simulink model "InnerOuter_Sim_newNav_flightgear_L2"  (Simulink 7.8)
settings: Solver=ode4  StartTime=0.0  StopTime=300  FixedStep=SampleT  RelTol=1e-3
InitFcn:
  | clc
  | innerOuterInit
  | launchFlightgear
values from neighbouring files (symbols this model uses):
  apSampleTime = 0.01    [innerOuterInit.m]
  FLIGHTGEAR_L2_RATE = 10    [launchFlightgear.m]
  SampleT = 0.005    [innerOuterInit.m]
  T = 0.01    [innerOuterInit.m]
undefined symbols (not defined in the file or in its folder): A1, Apolar, bankCommandLimit, baseHeight, BasePoint, baseTemp, CD0, chord, CL0, CLa, CLa_dot, Clb, ClDa, CLDe, CLDf, ClDr, clock, Clp, CLq, Clr, Cm0, Cma, CmDe, CmDf, Cmq, Cnb, CnDa, CnDr, Cnp, Cnr, compensatorOn, CYb, CYDr, da_failamp, da_failbias, da_failper, daL_fail, daR_fail, deg, DiscIntNeverNeededParam, dr_fail, dr_failamp, dr_failbias, dr_failper, Earth, elarm, Euler_0, F, gaind, getGSLocation, getWP, GS_location, Init_onlyOnce, Init_Reset, IPStar, ISA_g, Ixx, Iyy, Izz, L1OF ... (+38)
libraries: simulink x74, SLUGS_Library x41, aerolibconvert2 x24, dsPICdrivers x10, aerolibactuator x5, aerolibtransform2 x4, aerolibobsolete x3, dspmtrx3 x3, aerolibwind2 x2, aerolibfltsims x2, aerolibatmos2 x1, aerolibanimutils x1
(part 3 of 5)

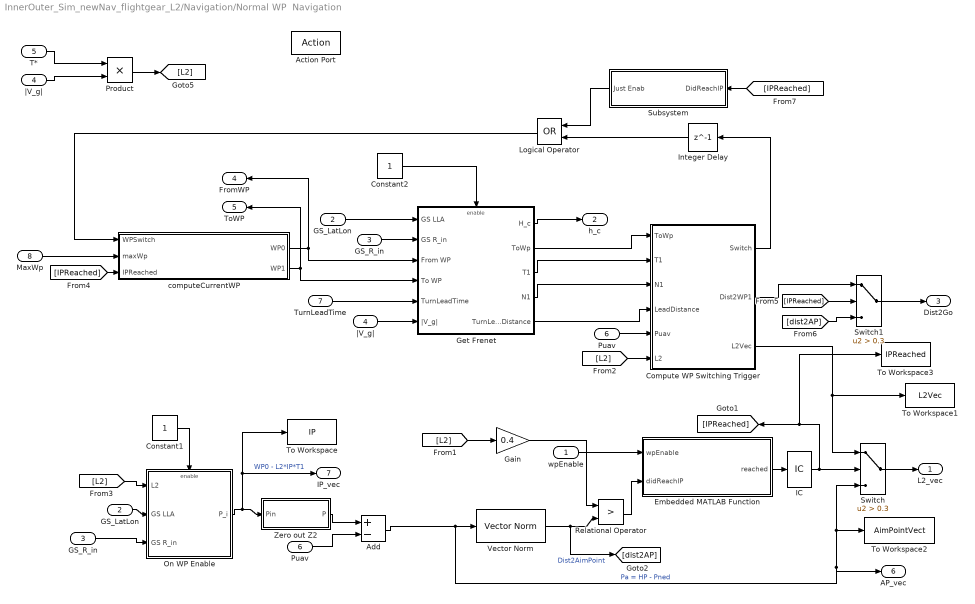
== system InnerOuter_Sim_newNav_flightgear_L2/Navigation/Normal WP  Navigation ==
  wpEnable : Inport
  GS_LatLon : Inport  Port=2
  GS_R_in : Inport  Port=3
  |V_g| : Inport  Port=4
  T* : Inport  Port=5
  Puav : Inport  Port=6
  TurnLeadTime : Inport  Port=7
  MaxWp : Inport  Port=8
  Action Port : ActionPort  ActionType=elseif
  Add : Sum  Inputs=+-
  Compute WP Switching Trigger : Subsystem
  Constant1 : Constant  OutDataTypeStr=boolean  SampleTime=0.01
  Constant2 : Constant  OutDataTypeStr=boolean  SampleTime=0.01
  Embedded MATLAB Function : MATLAB Function  TreatAsAtomicUnit=on
  "GS_LatLon " : InportShadow  Port=2
  "GS_R_in " : InportShadow  Port=3
  Gain : Gain  Gain=0.4
  Get Frenet : Subsystem
  IC : InitialCondition  Value=0
  Integer Delay : Delay  DelayLength=1  InitialCondition=1  InputProcessing=Inherited
  Logical Operator : Logic  Operator=OR  AllPortsSameDT=off  OutDataTypeStr=boolean
  On WP Enable : Subsystem  TreatAsAtomicUnit=on
  Product : Product  OutDataTypeStr=single  RndMeth=Zero
  "Puav " : InportShadow  Port=6
  Relational Operator : RelationalOperator  Operator=>  OutDataTypeStr=boolean
  Subsystem : Subsystem
  Switch : Switch  Criteria=u2 > Threshold  Threshold=0.3  ZeroCross=off
  Switch1 : Switch  Criteria=u2 > Threshold  Threshold=0.3  ZeroCross=off
  To Workspace : ToWorkspace  VariableName=IP  SampleTime=-1  SaveFormat=Array
  To Workspace1 : ToWorkspace  VariableName=L2Vec  SampleTime=-1  SaveFormat=Array
  To Workspace2 : ToWorkspace  VariableName=AimPointVect  SampleTime=-1  SaveFormat=Array
  To Workspace3 : ToWorkspace  VariableName=IPReached  SampleTime=-1  SaveFormat=Array
  Vector Norm : SLUGS_Library/Vector Norm
  Zero out Z2 : MATLAB Function  TreatAsAtomicUnit=on
  computeCurrentWP : MATLAB Function  TreatAsAtomicUnit=on
  "|V_g| " : InportShadow  Port=4
  L2_vec : Outport
  h_c : Outport  Port=2
  Dist2Go : Outport  Port=3
  FromWP : Outport  Port=4  InitialOutput=[1]
  ToWP : Outport  Port=5  InitialOutput=[2]
  AP_vec : Outport  Port=6
  IP_vec : Outport  Port=7
  wires:
  Get Frenet/1(H_c) -> h_c/1
  Constant2/1 -> Get Frenet/Enable
  Constant1/1 -> On WP Enable/Enable
  [IPReached] -> Subsystem/1(DidReachIP)
  Subsystem/1(Just Enab) -> Logical Operator/1
  Integer Delay/1 -> Logical Operator/2
  Logical Operator/1 -> computeCurrentWP/1(WPSwitch)
  [dist2AP] -> Switch1/3
  Switch1/1 -> Dist2Go/1
  Compute WP Switching Trigger/2(Dist2WP1) -> Switch1/1
  [IPReached] -> Switch1/2
  [IPReached] -> computeCurrentWP/3(IPReached)
  wpEnable/1 -> Embedded MATLAB Function/1(wpEnable)
  T*/1 -> Product/1
  |V_g|/1 -> Product/2
  Product/1 -> [L2]
  [L2] -> On WP Enable/1(L2)
  GS_LatLon/1 -> On WP Enable/2(GS LLA)
  GS_R_in/1 -> On WP Enable/3(GS R_in)
  On WP Enable/1(P_i) -> Zero out Z2/1(Pin), To Workspace/1, IP_vec/1  "WP0 - L2*IP*T1"
  Zero out Z2/1(P) -> Add/1
  Add/1 -> Vector Norm/1, Switch/3, To Workspace2/1, AP_vec/1  "Pa = HP - Pned"
  [L2] -> Gain/1
  Gain/1 -> Relational Operator/1
  Vector Norm/1 -> [dist2AP], Relational Operator/2  "Dist2AimPoint"
  Relational Operator/1 -> Embedded MATLAB Function/2(didReachIP)
  Switch/1 -> L2_vec/1
  Embedded MATLAB Function/1(reached) -> IC/1
  "GS_LatLon "/1 -> Get Frenet/1(GS LLA)
  "GS_R_in "/1 -> Get Frenet/2(GS R_in)
  Get Frenet/2(ToWp) -> Compute WP Switching Trigger/1(ToWp)
  Get Frenet/3(T1) -> Compute WP Switching Trigger/2(T1)
  Puav/1 -> Compute WP Switching Trigger/5(Puav)
  "Puav "/1 -> Add/2
  "|V_g| "/1 -> Get Frenet/6(|V_g|)
  TurnLeadTime/1 -> Get Frenet/5(TurnLeadTime)
  Get Frenet/5(TurnLeadDistance) -> Compute WP Switching Trigger/4(LeadDistance)
  Get Frenet/4(N1) -> Compute WP Switching Trigger/3(N1)
  Compute WP Switching Trigger/3(L2Vec) -> Switch/1, To Workspace1/1
  Compute WP Switching Trigger/1(Switch) -> Integer Delay/1
  computeCurrentWP/1(WP0) -> FromWP/1, Get Frenet/3(From WP)
  computeCurrentWP/2(WP1) -> ToWP/1, Get Frenet/4(To WP)
  MaxWp/1 -> computeCurrentWP/2(maxWp)
  [L2] -> Compute WP Switching Trigger/6(L2)
  IC/1 -> [IPReached], To Workspace3/1, Switch/2

== system InnerOuter_Sim_newNav_flightgear_L2/Navigation/RTB/Follow Mobile Navigation ==
  Mobile Location : Inport
  Follow Mobile? : Inport  Port=2
  MidLvl h_c : Inport  Port=3
  GS LatLon : Inport  Port=4
  GS R : Inport  Port=5
  Puav : Inport  Port=6
  Action Port : ActionPort  ActionType=then
  Compute Mobile Location : Subsystem  TreatAsAtomicUnit=on
  Constant : Constant  Value=[0 0 0]  OutDataTypeStr=single
  RTB : Constant  Value=0  OutDataTypeStr=uint8
  RTB1 : Constant  Value=0  OutDataTypeStr=uint8
  Simple Predictor : Subsystem
  Subtract : Sum  Inputs=+-
  Switch : Switch  Threshold=0.3
  To Workspace : ToWorkspace  VariableName=BP  SampleTime=-1  SaveFormat=Array
  Vector Norm : SLUGS_Library/Vector Norm
  Zero out Z1 : MATLAB Function  TreatAsAtomicUnit=on
  L2_vec : Outport
  h_c : Outport  Port=2
  Dist2Go : Outport  Port=3
  FromWP : Outport  Port=4  InitialOutput=[0]
  ToWP : Outport  Port=5  InitialOutput=[0]
  wires:
  RTB1/1 -> ToWP/1
  RTB/1 -> FromWP/1
  Vector Norm/1 -> Dist2Go/1
  Constant/1 -> Switch/3
  Compute Mobile Location/1(XYZ) -> Switch/1
  Follow Mobile?/1 -> Compute Mobile Location/Enable, Switch/2
  GS LatLon/1 -> Compute Mobile Location/2(GS LLA)
  GS R/1 -> Compute Mobile Location/3(GS R)
  Mobile Location/1 -> Compute Mobile Location/1("Lat, Lon")
  Simple Predictor/1(Predicted Bp) -> L2_vec/1
  Switch/1 -> Zero out Z1/1(Pin)
  Subtract/1 -> Vector Norm/1, Simple Predictor/1(Base Point), To Workspace/1
  Puav/1 -> Subtract/2
  Zero out Z1/1(P) -> Subtract/1
  MidLvl h_c/1 -> h_c/1

== system InnerOuter_Sim_newNav_flightgear_L2/Navigation/Recent Enable ==
  WP Fly : Inport
  Grab Upon Enable : Subsystem  TreatAsAtomicUnit=on
  IC1 : InitialCondition  Value=0
  IC2 : InitialCondition
  Subsystem : Subsystem
  WPEnable : Outport
  "GS, Lat Lon" : Outport  Port=2
  GS R_in : Outport  Port=3
  GS Alt (m) : Outport  Port=4
  wires:
  Grab Upon Enable/3(GS Altitude (m)) -> GS Alt (m)/1
  IC2/1 -> Grab Upon Enable/Enable
  IC1/1 -> Subsystem/1(WP Fly)
  Subsystem/1(Just Enab) -> IC2/1, WPEnable/1
  WP Fly/1 -> IC1/1
  Grab Upon Enable/1("GS, Lon, Lat") -> "GS, Lat Lon"/1
  Grab Upon Enable/2(GS R_in) -> GS R_in/1

== system InnerOuter_Sim_newNav_flightgear_L2/PT Unit (Vlad) /LPF the Euler and Construct Matrix ==
  Euler : Inport
  Euler Angles to  Direction Cosine Matrix : aerolibobsolete/Euler Angles to  Direction Cosine Matrix
  Terminator : Terminator
  "Tustin Lowpass, Auto Initial Condition1" : Subsystem  mask(Tustin1stOrderLowpassAutoInitialCondition){f=75, T=T}
      mask prompts: f "Lowpass Frequency"; T "Sample Time"
      mask help: Takes a 3db rolloff frequency (in Hz, NOT radians/s) and a sample time. Performs a symbolic Tustin conversion and implements in a discrete filter. The initial output of the filter is set by the first sample.
      mask Help: Enter the desired 3db rolloff frequency in Hz and the sample time. Initial conditions are sampled automatically.
      mask Display: fprintf('%.2f Hz lowpass',f)
  "Tustin Lowpass, Auto Initial Condition2" : Subsystem  mask(Tustin1stOrderLowpassAutoInitialCondition){f=75, T=T}
      mask prompts: f "Lowpass Frequency"; T "Sample Time"
      mask help: Takes a 3db rolloff frequency (in Hz, NOT radians/s) and a sample time. Performs a symbolic Tustin conversion and implements in a discrete filter. The initial output of the filter is set by the first sample.
      mask Help: Enter the desired 3db rolloff frequency in Hz and the sample time. Initial conditions are sampled automatically.
      mask Display: fprintf('%.2f Hz lowpass',f)
  "Tustin Lowpass, Auto Initial Condition3" : Subsystem  mask(Tustin1stOrderLowpassAutoInitialCondition){f=75, T=T}
      mask prompts: f "Lowpass Frequency"; T "Sample Time"
      mask help: Takes a 3db rolloff frequency (in Hz, NOT radians/s) and a sample time. Performs a symbolic Tustin conversion and implements in a discrete filter. The initial output of the filter is set by the first sample.
      mask Help: Enter the desired 3db rolloff frequency in Hz and the sample time. Initial conditions are sampled automatically.
      mask Display: fprintf('%.2f Hz lowpass',f)
  "[a b c]" : Demux  Outputs=3
  myMux Fun5 : MATLAB Function  TreatAsAtomicUnit=on
  Rfg2b : Outport
  wires:
  myMux Fun5/1(y) -> Terminator/1
  Euler/1 -> Euler Angles to  Direction Cosine Matrix/1, "[a b c]"/1
  "[a b c]"/3 -> "Tustin Lowpass, Auto Initial Condition3"/1(In1)
  "[a b c]"/2 -> "Tustin Lowpass, Auto Initial Condition1"/1(In1)
  "[a b c]"/1 -> "Tustin Lowpass, Auto Initial Condition2"/1(In1)
  "Tustin Lowpass, Auto Initial Condition3"/1(Out1) -> myMux Fun5/3(u3)
  "Tustin Lowpass, Auto Initial Condition1"/1(Out1) -> myMux Fun5/2(u2)
  "Tustin Lowpass, Auto Initial Condition2"/1(Out1) -> myMux Fun5/1(u1)
  Euler Angles to  Direction Cosine Matrix/1 -> Rfg2b/1

== system InnerOuter_Sim_newNav_flightgear_L2/Simple Car Model/Heading/Speed to Velocity ==
  Heading : Inport
  Speed : Inport  Port=2
  Add : Sum  Inputs=+-
  Angle Conversion : aerolibconvert2/Angle Conversion  IU=deg  OU=rad
  Divide : Product
  Divide1 : Product
  Low pass the  change of direction : Subsystem  mask(Tustin1stOrderLowpassAutoInitialCondition){f=0.05, T=apSampleTime}
      mask prompts: f "Lowpass Frequency"; T "Sample Time"
      mask help: Takes a 3db rolloff frequency (in Hz, NOT radians/s) and a sample time. Performs a symbolic Tustin conversion and implements in a discrete filter. The initial output of the filter is set by the first sample.
      mask Help: Enter the desired 3db rolloff frequency in Hz and the sample time. Initial conditions are sampled automatically.
      mask Display: fprintf('%.2f Hz lowpass',f)
  Mux : Mux  Inputs=3
  Rate Transition1 : RateTransition  OutPortSampleTime=apSampleTime
  Rate Transition2 : RateTransition  OutPortSampleTime=apSampleTime
  Speed1 : Constant  Value=0
  Speed2 : Constant  Value=450*pi/180  SampleTime=0.01
  Trigonometric Function : Trigonometry  Operator=cos
  Trigonometric Function1 : Trigonometry
  Velocity : Outport
  wires:
  Speed1/1 -> Mux/3
  Speed2/1 -> Add/1
  Add/1 -> Trigonometric Function/1, Trigonometric Function1/1  "alpha"
  Trigonometric Function/1 -> Divide/1
  Speed/1 -> Rate Transition2/1
  Divide/1 -> Mux/1
  Angle Conversion/1 -> Add/2
  Divide1/1 -> Mux/2
  Trigonometric Function1/1 -> Divide1/2
  Low pass the  change of direction/1(Out1) -> Angle Conversion/1
  Heading/1 -> Rate Transition1/1
  Mux/1 -> Velocity/1
  Rate Transition1/1 -> Low pass the  change of direction/1(In1)
  Rate Transition2/1 -> Divide1/1, Divide/2

== system InnerOuter_Sim_newNav_flightgear_L2/Simple Car Model/Simple Car Model ==
  Velocity : Inport
  Constant13 : Constant  Value=BasePoint  OutDataTypeStr=single
  Data Type Conversion : DataTypeConversion  OutDataTypeStr=single
  Data Type Conversion1 : DataTypeConversion  OutDataTypeStr=single
  Discrete-Time Integrator : DiscreteIntegrator  InitialConditionSource=external  SampleTime=0.01  ICPrevOutput=DiscIntNeverNeededParam  ICPrevScaledInput=DiscIntNeverNeededParam
  p_cg : Outport
  wires:
  Velocity/1 -> Data Type Conversion1/1
  Constant13/1 -> Discrete-Time Integrator/2
  Discrete-Time Integrator/1 -> Data Type Conversion/1
  Data Type Conversion/1 -> p_cg/1
  Data Type Conversion1/1 -> Discrete-Time Integrator/1

== system InnerOuter_Sim_newNav_flightgear_L2/6DOF Model/Plant/6-DOF EOM ==
  "[F,M]" : Inport
  Vb Corr : Inport  Port=2
  Angular Rates : Integrator  InitialCondition=PQR_0'
  Demux1 : Demux  Outputs=2
  Euler Angles : Integrator  InitialCondition=Euler_0
  Get Euler Dot : Subsystem
      mask Display:
      | port_label('input', 1, 'p, q, r')
      | port_label('input', 2, 'Euler')
      | port_label('output', 1, 'Euler_dot')
  Mux : Mux  Inputs=[3;3]
  NED2NEU : Gain  Gain=[1 0 0;0 1 0;0 0 -1]  Multiplication=Matrix(K*u)  SaturateOnIntegerOverflow=on  OutDataTypeStr=Inherit: Same as input  ParamDataTypeStr=Inherit: Same as input
  Position : Integrator  InitialCondition=Pos_0'
  RB2L * Vb : Product  Multiplication=Matrix(*)  SaturateOnIntegerOverflow=on  InputSameDT=on  OutDataTypeStr=Inherit: Same as first input
  RB2LTP : Subsystem
  Velocities Body : Integrator  InitialCondition=Vb_0'
  "[V1,2,3,W1,2,3]" : Subsystem
  X,Y,Z (LTP) : Outport
  "Vx, Vy, Vz" : Outport  Port=2
  Euler : Outport  Port=3
  "p, q, r" : Outport  Port=4
  Vb : Outport  Port=5
  Ab meas : Outport  Port=6
  Euler_dot : Outport  Port=7
  wires:
  "[V1,2,3,W1,2,3]"/1("Acc_meas ") -> Ab meas/1
  Euler Angles/1 -> "[V1,2,3,W1,2,3]"/2(Euler), Get Euler Dot/2(Euler), Euler/1, RB2LTP/1(Euler)
  Demux1/1 -> Velocities Body/1
  "[V1,2,3,W1,2,3]"/2(V*dot) -> Demux1/1
  Demux1/2 -> Angular Rates/1
  "[F,M]"/1 -> "[V1,2,3,W1,2,3]"/1("[F ; M]")
  RB2LTP/1(Rot) -> RB2L * Vb/1
  Velocities Body/1 -> Vb/1, RB2L * Vb/2
  Mux/1 -> "[V1,2,3,W1,2,3]"/3(V*)
  Position/1 -> X,Y,Z (LTP)/1
  Angular Rates/1 -> Get Euler Dot/1(p,q,r), Mux/2, "p, q, r"/1
  RB2L * Vb/1 -> NED2NEU/1, "Vx, Vy, Vz"/1  "NED"
  NED2NEU/1 -> Position/1
  Get Euler Dot/1(Euler_dot) -> Euler Angles/1, Euler_dot/1
  Vb Corr/1 -> Mux/1

== system InnerOuter_Sim_newNav_flightgear_L2/6DOF Model/Plant/Engine Model ==
  dt : Inport
  Vmag : Inport  Port=2
  Constant4 : Constant  Value=0
  Get To1 : Subsystem
  Mux : Mux  Inputs=2
  Mux1 : Mux  Inputs=3
  Thrust Available (lbs) : Fcn  Expr=u(1) - 0.047*sqrt(u(1))*u(2)
  kg2N : Gain  Gain=ISA_g  SaturateOnIntegerOverflow=on  OutDataTypeStr=Inherit: Same as input  ParamDataTypeStr=Inherit: Same as input
  lbs2kg : Gain  Gain=0.45359237  SaturateOnIntegerOverflow=on  OutDataTypeStr=Inherit: Same as input  ParamDataTypeStr=Inherit: Same as input
  Thrust : Outport
  wires:
  dt/1 -> Get To1/1(dt)
  Get To1/1(To) -> Mux/1
  Mux/1 -> Thrust Available (lbs)/1
  Thrust Available (lbs)/1 -> lbs2kg/1
  Vmag/1 -> Mux/2
  Mux1/1 -> Thrust/1
  lbs2kg/1 -> kg2N/1
  Constant4/1 -> Mux1/2, Mux1/3
  kg2N/1 -> Mux1/1

== system InnerOuter_Sim_newNav_flightgear_L2/6DOF Model/Plant/Forces and Moments ==
  "Wind {E}" : Inport
  Rho : Inport  Port=2
  "de, deg" : Inport  Port=3
  daL,deg : Inport  Port=4
  daR,deg : Inport  Port=5
  "dr, deg" : Inport  Port=6
  "df, deg" : Inport  Port=7
  "Vx, Vy, Vz " : Inport  Port=8
  Euler : Inport  Port=9  PortDimensions=3
  p,q,r : Inport  Port=10
  Alpha/Beta : Subsystem
  Body Frame F & M : Subsystem
  Get Grav Force in Body : Subsystem
  Gravitational Force : Constant  Value=[0 0 mass*ISA_g]  VectorParams1D=off
  NED(u)2b : Subsystem
  Sum : Sum  Inputs=|++  SaturateOnIntegerOverflow=on
  Vair : Sum  Inputs=+-  SaturateOnIntegerOverflow=on  InputSameDT=on  OutDataTypeStr=Inherit: Same as first input
  Airspeed : Outport
  Forces : Outport  Port=2
  Moments : Outport  Port=3
  Vb Corr : Outport  Port=4
  q : Outport  Port=5
  wires:
  Get Grav Force in Body/1(Grav Force (Body)) -> Sum/2
  Alpha/Beta/5(q) -> q/1
  "Vx, Vy, Vz "/1 -> Vair/1
  Vair/1 -> NED(u)2b/1(V w)
  Euler/1 -> NED(u)2b/2(Euler), Get Grav Force in Body/1(Euler)
  Rho/1 -> Alpha/Beta/2(Rho)
  NED(u)2b/1(Vb Corr) -> Alpha/Beta/1("Vx, Vy, Vz (Body)"), Vb Corr/1
  Body Frame F & M/2(M_b) -> Moments/1
  Gravitational Force/1 -> Get Grav Force in Body/2(Grav Force)
  Body Frame F & M/1(F_b) -> Sum/1
  Sum/1 -> Forces/1
  Alpha/Beta/3(qS) -> Body Frame F & M/3(qs)
  Alpha/Beta/4(Speed) -> Body Frame F & M/4(Airspeed), Airspeed/1
  "df, deg"/1 -> Body Frame F & M/9("df, deg")
  p,q,r/1 -> Body Frame F & M/10(p,q,r)
  Alpha/Beta/2("beta, deg") -> Body Frame F & M/2("Beta, deg")
  "dr, deg"/1 -> Body Frame F & M/8("dr, deg")
  daL,deg/1 -> Body Frame F & M/6("daL, deg")
  Alpha/Beta/1("alpha, deg") -> Body Frame F & M/1("Alpha, deg")
  "de, deg"/1 -> Body Frame F & M/5("de, deg")
  "Wind {E}"/1 -> Vair/2
  daR,deg/1 -> Body Frame F & M/7("daR, deg")

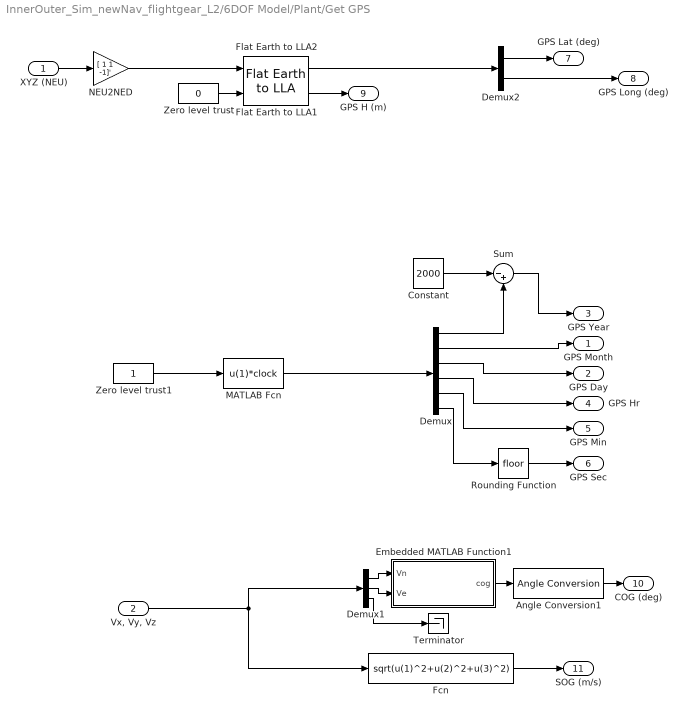
== system InnerOuter_Sim_newNav_flightgear_L2/6DOF Model/Plant/Get GPS ==
  XYZ (NEU) : Inport
  "Vx, Vy, Vz" : Inport  Port=2
  Angle Conversion1 : aerolibconvert2/Angle Conversion  IU=rad  OU=deg
  Constant : Constant  Value=2000
  Demux : Demux  Outputs=6
  Demux1 : Demux  Outputs=3
  Demux2 : Demux  Outputs=2
  Embedded MATLAB Function1 : MATLAB Function  TreatAsAtomicUnit=on
  Fcn : Fcn  Expr=sqrt(u(1)^2+u(2)^2+u(3)^2)
  Flat Earth to LLA1 : aerolibtransform2/Flat Earth to LLA  units=Metric (MKS)  ptype=Earth (WGS84)  F=1/298.257223563  R=6378137  LL0=GS_location(2:3)  psi=0
  Flat Earth to LLA2 : aerolibtransform2/Flat Earth to LLA  units=Metric (MKS)  ptype=Earth (WGS84)  F=1/298.257223563  R=6378137  LL0=GS_location(2:3)  psi=0
  MATLAB Fcn : MATLABFcn  MATLABFcn=u(1)*clock  OutputSignalType=real  SampleTime=SampleT
  NEU2NED : Gain  Gain=[ 1 1 -1]'  SaturateOnIntegerOverflow=on  OutDataTypeStr=Inherit: Same as input  ParamDataTypeStr=Inherit: Same as input
  Rounding Function : Rounding
  Sum : Sum  Inputs=|-+
  Terminator : Terminator
  Zero level trust : Constant  Value=0  SampleTime=SampleT
  Zero level trust1 : Constant  SampleTime=SampleT
  GPS Month : Outport
  GPS Day : Outport  Port=2
  GPS Year : Outport  Port=3
  GPS Hr : Outport  Port=4
  GPS Min : Outport  Port=5
  GPS Sec : Outport  Port=6
  GPS Lat (deg) : Outport  Port=7
  GPS Long (deg) : Outport  Port=8
  GPS H (m) : Outport  Port=9
  COG (deg) : Outport  Port=10
  SOG (m/s) : Outport  Port=11
  wires:
  NEU2NED/1 -> Flat Earth to LLA2/1
  Zero level trust/1 -> Flat Earth to LLA2/2
  XYZ (NEU)/1 -> NEU2NED/1
  Flat Earth to LLA2/1 -> Demux2/1
  Flat Earth to LLA2/2 -> GPS H (m)/1
  Zero level trust1/1 -> MATLAB Fcn/1
  MATLAB Fcn/1 -> Demux/1
  Demux/2 -> GPS Month/1
  Demux/3 -> GPS Day/1
  Demux/4 -> GPS Hr/1
  Demux/5 -> GPS Min/1
  Demux/6 -> Rounding Function/1
  Rounding Function/1 -> GPS Sec/1
  Demux2/1 -> GPS Lat (deg)/1
  Demux2/2 -> GPS Long (deg)/1
  Fcn/1 -> SOG (m/s)/1
  Demux1/1 -> Embedded MATLAB Function1/1(Vn)
  Demux1/2 -> Embedded MATLAB Function1/2(Ve)
  "Vx, Vy, Vz"/1 -> Demux1/1, Fcn/1
  Embedded MATLAB Function1/1(cog) -> Angle Conversion1/1
  Angle Conversion1/1 -> COG (deg)/1
  Demux/1 -> Sum/2
  Constant/1 -> Sum/1
  Sum/1 -> GPS Year/1
  Demux1/3 -> Terminator/1

== system InnerOuter_Sim_newNav_flightgear_L2/6DOF Model/Plant/ISA Atmosphere & Winds ==
  "X, Y, Z" : Inport
  Euler : Inport  Port=2
  Wind On : Inport  Port=3
  Airspeed : Inport  Port=4
  Add : Sum  Inputs=2
  Constant : Constant  Value=[ 0 0 0]
  Dryden Wind Turbulence Model  (Discrete (+q -r)) : aerolibwind2/Dryden Wind Turbulence Model  (Continuous (+q -r))  units=Metric (MKS)  spec=MIL-F-8785C  model=Discrete Dryden (+q -r)  W20=windBase*0.3  Wdeg=windDirTurb  TurbProb=10^-2 - Light  L_high=533.4  Wingspan=span  ts=0.005  Seed=[23341 23342 23343 23344]  T_on=on
  Euler Angles to  Direction Cosine Matrix1 : aerolibobsolete/Euler Angles to  Direction Cosine Matrix
  Get Z : Selector  InputPortWidth=3  IndexOptions=Index vector (dialog)  Indices=[3]  OutputSizes=[(-2)]
  Horizontal Wind Model : aerolibwind2/Horizontal Wind Model  units=Metric (MKS)  Vw_source=Internal  Vwind=windBase  W_source=Internal  Wdeg=windDirHor
  ISA Atmosphere Model1 : aerolibatmos2/ISA Atmosphere Model  custom=off  g=9.80665  gamma=1.4  R=287.0531  L=0.0065  h_trop=11000  h_strat=20000  rho0=1.225  P0=101325  T0=288.15
  Reduce Z Wind : Gain  Gain=[1 1 0.1]
  Rotate to E Frame : Product  Multiplication=Matrix(*)
  Scope : Scope
      settings: YMin=-1  YMax=13  SaveName=windData  DataFormat=Array
  Switch : Switch  Criteria=u2 > Threshold  Threshold=0.3
  Terminator1 : Terminator
  Transpose : dspmtrx3/Transpose  Hermitian=off  overflowFlag=off
  Unit Delay : UnitDelay  SampleTime=-1
  Rho : Outport
  "Wind, {E}" : Outport  Port=2
  AirPressure (Pa) : Outport  Port=3
  OAT (K) : Outport  Port=4
  wires:
  "X, Y, Z"/1 -> Get Z/1
  Get Z/1 -> ISA Atmosphere Model1/1, Dryden Wind Turbulence Model  (Discrete (+q -r))/1
  ISA Atmosphere Model1/4 -> Rho/1
  ISA Atmosphere Model1/1 -> OAT (K)/1
  ISA Atmosphere Model1/2 -> Terminator1/1
  ISA Atmosphere Model1/3 -> AirPressure (Pa)/1
  Euler/1 -> Euler Angles to  Direction Cosine Matrix1/1
  Euler Angles to  Direction Cosine Matrix1/1 -> Dryden Wind Turbulence Model  (Discrete (+q -r))/3, Horizontal Wind Model/1, Transpose/1  "RECEF2B"
  Airspeed/1 -> Unit Delay/1
  Add/1 -> Switch/1
  Unit Delay/1 -> Dryden Wind Turbulence Model  (Discrete (+q -r))/2
  Horizontal Wind Model/1 -> Add/2
  Switch/1 -> Rotate to E Frame/2
  Wind On/1 -> Switch/2
  Constant/1 -> Switch/3
  Transpose/1 -> Rotate to E Frame/1
  Rotate to E Frame/1 -> "Wind, {E}"/1, Scope/1
  Dryden Wind Turbulence Model  (Discrete (+q -r))/1 -> Reduce Z Wind/1
  Reduce Z Wind/1 -> Add/1

== system InnerOuter_Sim_newNav_flightgear_L2/6DOF Model/Plant/Magnetometer ==
  Euler : Inport
  LTP2B : dspmtrx3/Transpose  Hermitian=off  overflowFlag=off
  Mag Field in nT source:  http://www.ngdc.noaa.gov/geomagmodels/struts/calcIGRFWMM : Constant  Value=magField
  Product : Product  Multiplication=Matrix(*)  RndMeth=Zero
  RB2LTP : Subsystem
  "Mag, nT" : Outport
  wires:
  RB2LTP/1(Rot) -> LTP2B/1
  LTP2B/1 -> Product/1
  Mag Field in nT source:  http://www.ngdc.noaa.gov/geomagmodels/struts/calcIGRFWMM/1 -> Product/2
  Euler/1 -> RB2LTP/1(Euler)
  Product/1 -> "Mag, nT"/1

== system InnerOuter_Sim_newNav_flightgear_L2/6DOF Model/Plant/[0, pi] Wrap Around ==
  Euler : Inport
  Compare To Zero : simulink/Logic and Bit Operations/Compare To Zero  relop=>=  OutDataTypeStr=uint8  ZeroCross=off
  Logical Operator : Logic  Operator=NOT  AllPortsSameDT=off  OutDataTypeStr=boolean
  Merge : Merge
  Mux2 : Mux  Inputs=2
  Negative Yaw : Subsystem
  Positive Yaw : Subsystem
  Selector1 : Selector  InputPortWidth=3  IndexOptions=Index vector (dialog)  Indices=[1 2]  OutputSizes=1
  Selector2 : Selector  InputPortWidth=3  IndexOptions=Index vector (dialog)  Indices=[3]  OutputSizes=1
  Euler-Wrapped : Outport
  wires:
  Euler/1 -> Selector2/1, Selector1/1
  Selector1/1 -> Mux2/1
  Mux2/1 -> Euler-Wrapped/1
  Selector2/1 -> Compare To Zero/1, Positive Yaw/1(yaw), Negative Yaw/1(yaw)
  Compare To Zero/1 -> Positive Yaw/Enable, Logical Operator/1
  Logical Operator/1 -> Negative Yaw/Enable
  Merge/1 -> Mux2/2
  Positive Yaw/1(yaw_wr) -> Merge/1
  Negative Yaw/1(yaw_wr) -> Merge/2

== system InnerOuter_Sim_newNav_flightgear_L2/6DOF Model/Split Ailerons And Introduce Failures/Aileron Flaping Failure ==
  Pulse Generator1 : DiscretePulseGenerator  PulseType=Time based  Amplitude=da_failamp  Period=da_failper  PulseWidth=50
  Vair2 : Sum  Inputs=+++  SaturateOnIntegerOverflow=on  InputSameDT=on  OutDataTypeStr=Inherit: Same as first input
  da_failbias : Constant  Value=da_failbias
  da_failbias1 : Constant  Value=0
  "da, Fail, deg" : Outport
  wires:
  Pulse Generator1/1 -> Vair2/1
  da_failbias/1 -> Vair2/2
  da_failbias1/1 -> Vair2/3
  Vair2/1 -> "da, Fail, deg"/1

== system InnerOuter_Sim_newNav_flightgear_L2/6DOF Model/Split Ailerons And Introduce Failures/Rudder Failure ==
  Pulse Generator1 : DiscretePulseGenerator  PulseType=Time based  Amplitude=dr_failamp  Period=dr_failper  PulseWidth=50
  Vair2 : Sum  Inputs=+++  SaturateOnIntegerOverflow=on  InputSameDT=on  OutDataTypeStr=Inherit: Same as first input
  da_failbias : Constant  Value=dr_failbias
  da_failbias1 : Constant  Value=0
  "da, Fail, deg" : Outport
  wires:
  Vair2/1 -> "da, Fail, deg"/1
  da_failbias1/1 -> Vair2/3
  da_failbias/1 -> Vair2/2
  Pulse Generator1/1 -> Vair2/1

== system InnerOuter_Sim_newNav_flightgear_L2/BaroTest/Initial Baro Bias/Low Pass8 ==
  In1 : Inport
  Discrete Zero-Pole : DiscreteZeroPole  Zeros=zerosd  Poles=polesd  Gain=gaind  SampleTime=SampleTime
  Out1 : Outport
  wires:
  In1/1 -> Discrete Zero-Pole/1
  Discrete Zero-Pole/1 -> Out1/1

== system InnerOuter_Sim_newNav_flightgear_L2/L1 Output Feedback Controller With  Projection Operator/Control  Law/Compute Coef ==
  a : Inport
  Enable : EnablePort
  -T : Gain  Gain=-apSampleTime  SampleTime=apSampleTime
  1-c : Sum  Inputs=-+  OutDataTypeStr=single  SampleTime=apSampleTime
  Constant : Constant
  Subsystem11 : Subsystem  AncestorBlock=SLUGS_Library/Subsystem11
  b : Outport
  c : Outport  Port=2
  wires:
  a/1 -> -T/1
  1-c/1 -> b/1
  Constant/1 -> 1-c/2
  Subsystem11/1(exp(u)) -> c/1, 1-c/1  "c"
  -T/1 -> Subsystem11/1(u)

== system InnerOuter_Sim_newNav_flightgear_L2/L1 Output Feedback Controller With  Projection Operator/Control  Law/Detect Change ==
  Data : Inport
  Abs1 : Abs  SampleTime=apSampleTime
  Difference1 : simulink/Discrete/Difference  ICPrevInput=0.0  InputProcessing=Inherited  OutMin=[]  OutMax=[]  OutDataType=sfix(16)  OutScaling=2^-10  DoSatur=off
  Saturation1 : Saturate  UpperLimit=1  LowerLimit=0  SampleTime=apSampleTime
  change? : Outport
  wires:
  Saturation1/1 -> change?/1
  Data/1 -> Difference1/1
  Abs1/1 -> Saturation1/1
  Difference1/1 -> Abs1/1

== system InnerOuter_Sim_newNav_flightgear_L2/L1 Output Feedback Controller With  Projection Operator/Projection Operator/Enabled Subsystem ==
  In1 : Inport
  Enable : EnablePort
  Out1 : Outport
  wires:
  In1/1 -> Out1/1

== system InnerOuter_Sim_newNav_flightgear_L2/L1 Output Feedback Controller With  Projection Operator/Projection Operator/Enabled Subsystem1 ==
  y : Inport
  f_the : Inport  Port=2
  grad : Inport  Port=3
  Enable : EnablePort
  Constant : Constant  OutDataTypeStr=single
  Divide1 : Product  OutDataTypeStr=single
  Divide2 : Product  OutDataTypeStr=single
  Sign : Signum
  Subtract : Sum  Inputs=+-  OutDataTypeStr=single
  Out1 : Outport
  wires:
  Divide2/1 -> Out1/1
  y/1 -> Divide2/1
  Subtract/1 -> Divide2/2
  f_the/1 -> Divide1/1
  Constant/1 -> Subtract/1
  Sign/1 -> Divide1/2
  grad/1 -> Sign/1
  Divide1/1 -> Subtract/2

== system InnerOuter_Sim_newNav_flightgear_L2/L1 Output Feedback Controller With  Projection Operator/Projection Operator/Enabled Subsystem2 ==
  y : Inport
  f_the : Inport  Port=2
  grad : Inport  Port=3
  Enable : EnablePort
  Constant : Constant  OutDataTypeStr=single
  Divide1 : Product  OutDataTypeStr=single
  Divide2 : Product  OutDataTypeStr=single
  Sign : Signum
  Subtract : Sum  Inputs=+-  OutDataTypeStr=single
  Out1 : Outport
  wires:
  Divide1/1 -> Subtract/2
  grad/1 -> Sign/1
  Sign/1 -> Divide1/2
  Constant/1 -> Subtract/1
  f_the/1 -> Divide1/1
  Subtract/1 -> Divide2/2
  y/1 -> Divide2/1
  Divide2/1 -> Out1/1

== system InnerOuter_Sim_newNav_flightgear_L2/L1 Output Feedback Controller With  Projection Operator/Projection Operator/F(theta) ==
  Theta Max : Inport
  Eps 0 : Inport  Port=2
  Theta : Inport  Port=3
  Constant : Constant  Value=2  OutDataTypeStr=single
  Divide : Product  OutDataTypeStr=single
  Divide1 : Product  OutDataTypeStr=single
  Divide2 : Product  OutDataTypeStr=single
  Divide3 : Product  Inputs=*/  OutDataTypeStr=single
  Divide4 : Product  Inputs=/**  OutDataTypeStr=single
  Subtract : Sum  Inputs=+-  OutDataTypeStr=single
  "Theta " : InportShadow  Port=3
  f_theta : Outport
  dif_f_theta : Outport  Port=2
  wires:
  Divide4/1 -> dif_f_theta/1
  "Theta "/1 -> Divide4/2
  Constant/1 -> Divide4/3
  Divide3/1 -> f_theta/1
  Divide2/1 -> Divide4/1, Divide3/2
  Subtract/1 -> Divide3/1
  Eps 0/1 -> Divide2/2
  Divide1/1 -> Divide2/1, Subtract/2
  Divide/1 -> Subtract/1
  Theta Max/1 -> Divide1/1, Divide1/2
  Theta/1 -> Divide/2, Divide/1

== system InnerOuter_Sim_newNav_flightgear_L2/L1 Output Feedback Controller With  Projection Operator/State Predictor/Compute Coef ==
  a : Inport
  Enable : EnablePort
  -T : Gain  Gain=-apSampleTime  SampleTime=apSampleTime
  1-c : Sum  Inputs=-+  OutDataTypeStr=single
  Constant : Constant
  Subsystem11 : Subsystem  AncestorBlock=SLUGS_Library/Subsystem11
  b : Outport
  c : Outport  Port=2
  wires:
  -T/1 -> Subsystem11/1(u)
  Subsystem11/1(exp(u)) -> 1-c/1, c/1  "c"
  Constant/1 -> 1-c/2
  1-c/1 -> b/1
  a/1 -> -T/1

== system InnerOuter_Sim_newNav_flightgear_L2/L1 Output Feedback Controller With  Projection Operator/State Predictor/Detect Change ==
  Data : Inport
  Abs1 : Abs  SampleTime=apSampleTime
  Difference1 : simulink/Discrete/Difference  ICPrevInput=0.0  InputProcessing=Inherited  OutMin=[]  OutMax=[]  OutDataType=sfix(16)  OutScaling=2^-10  DoSatur=off
  Saturation1 : Saturate  UpperLimit=1  LowerLimit=0  SampleTime=apSampleTime
  change? : Outport
  wires:
  Difference1/1 -> Abs1/1
  Abs1/1 -> Saturation1/1
  Data/1 -> Difference1/1
  Saturation1/1 -> change?/1

== system InnerOuter_Sim_newNav_flightgear_L2/L1 Output Feedback Controller With  Projection Operator/Trapezoidal Integrator/Protect NaNs ==
  In1 : Inport
  Integer Delay3 : Delay  DelayLength=1  InputProcessing=Inherited  SampleTime=T
  Relational Operator2 : RelationalOperator  Operator===  OutDataTypeStr=uint(8)
  Switch3 : Switch  Criteria=u2 > Threshold  Threshold=0.3  SampleTime=.01
  Out1 : Outport
  wires:
  Integer Delay3/1 -> Switch3/3
  Switch3/1 -> Out1/1, Integer Delay3/1
  In1/1 -> Relational Operator2/2, Relational Operator2/1, Switch3/1
  Relational Operator2/1 -> Switch3/2

== system InnerOuter_Sim_newNav_flightgear_L2/L1 Output Feedback Controller With  Projection Operator/Trapezoidal Integrator/Protect NaNs1 ==
  In1 : Inport
  Integer Delay3 : Delay  DelayLength=1  InputProcessing=Inherited  SampleTime=T
  Relational Operator2 : RelationalOperator  Operator===  OutDataTypeStr=uint(8)
  Switch3 : Switch  Criteria=u2 > Threshold  Threshold=0.3  SampleTime=.01
  Out1 : Outport
  wires:
  Relational Operator2/1 -> Switch3/2
  In1/1 -> Switch3/1, Relational Operator2/1, Relational Operator2/2
  Switch3/1 -> Integer Delay3/1, Out1/1
  Integer Delay3/1 -> Switch3/3

== system InnerOuter_Sim_newNav_flightgear_L2/Navigation/Circle Navigation/Get SP Location ==
  GS LLA : Inport
  GS R_in : Inport  Port=2
  ISR Location : Inport  Port=3
  Demux : Demux  Outputs=3
  Geod2LTP : SLUGS_Library/Navigation/Geod2LTP
  Integer Delay1 : Delay  DelayLength=1  InputProcessing=Inherited
  Selector : Selector  InputPortWidth=3  IndexOptions=Index vector (dialog)  Indices=[3]  OutputSizes=1
  Zero out Z2 : MATLAB Function  TreatAsAtomicUnit=on
  Hc : Outport
  SP : Outport  Port=2
  wires:
  Integer Delay1/1 -> Hc/1
  Selector/1 -> Integer Delay1/1
  Zero out Z2/1(P) -> SP/1
  Geod2LTP/1 -> Selector/1, Zero out Z2/1(Pin)
  GS LLA/1 -> Geod2LTP/1
  Demux/3 -> Geod2LTP/5
  Demux/2 -> Geod2LTP/4
  Demux/1 -> Geod2LTP/3
  GS R_in/1 -> Geod2LTP/2
  ISR Location/1 -> Demux/1

== system InnerOuter_Sim_newNav_flightgear_L2/Navigation/Circle Navigation/Inside the Circle,  Keep Straight until  intersection ==
  ISR Loc : Inport
  R : Inport  Port=2
  Puav : Inport  Port=3
  Action Port : ActionPort  ActionType=elseif
  Compute Head of Circle : MATLAB Function  TreatAsAtomicUnit=on
  RTB1 : Constant  OutDataTypeStr=uint8
  Subtract : Sum  Inputs=+-  OutDataTypeStr=single
  L2 Vec : Outport
  Mode : Outport  Port=2
  wires:
  RTB1/1 -> Mode/1
  R/1 -> Compute Head of Circle/1(R)
  ISR Loc/1 -> Compute Head of Circle/2(ISR)
  Compute Head of Circle/1(topCoord) -> Subtract/1
  Puav/1 -> Subtract/2
  Subtract/1 -> L2 Vec/1

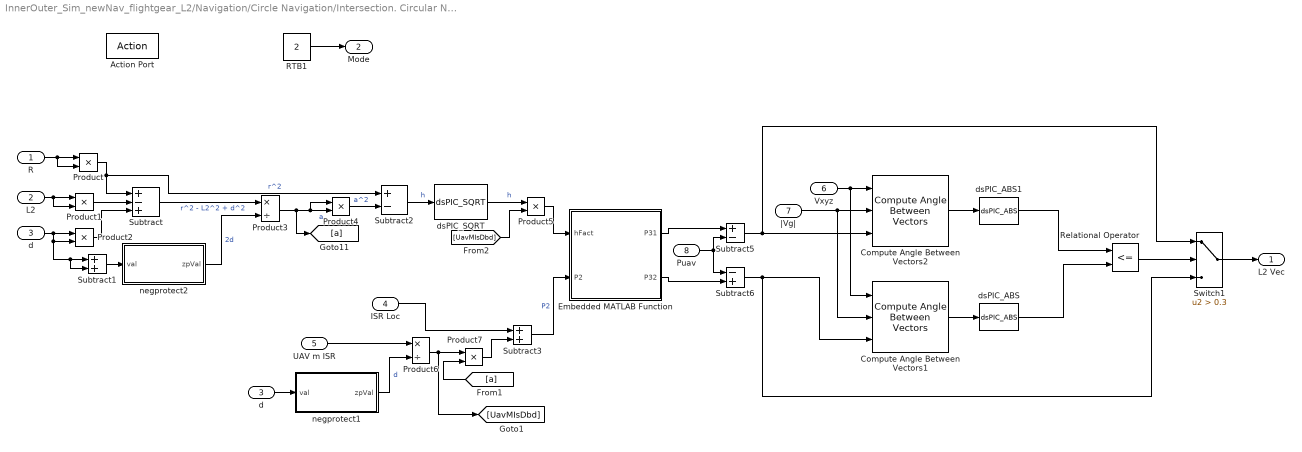
== system InnerOuter_Sim_newNav_flightgear_L2/Navigation/Circle Navigation/Intersection. Circular Navigation ==
  R : Inport
  L2 : Inport  Port=2
  d : Inport  Port=3
  ISR Loc : Inport  Port=4
  UAV m ISR : Inport  Port=5
  Vxyz : Inport  Port=6
  |Vg| : Inport  Port=7
  Puav : Inport  Port=8
  Action Port : ActionPort  ActionType=else
  Compute Angle Between Vectors1 : SLUGS_Library/Compute Angle Between Vectors
  Compute Angle Between Vectors2 : SLUGS_Library/Compute Angle Between Vectors
  Embedded MATLAB Function : MATLAB Function  TreatAsAtomicUnit=on
  Product{,1..2,4..5,7} (6 alike) : Product  RndMeth=Zero
  Product3 : Product  Inputs=*/  RndMeth=Zero
  Product6 : Product  Inputs=*/  RndMeth=Zero
  RTB1 : Constant  Value=2  OutDataTypeStr=uint8
  Relational Operator : RelationalOperator  Operator=<=  OutDataTypeStr=boolean
  Subtract : Sum  Inputs=+-+
  Subtract1 : Sum  Inputs=2
  Subtract2 : Sum  Inputs=+-
  Subtract3 : Sum  Inputs=2
  Subtract5 : Sum  Inputs=+-
  Subtract6 : Sum  Inputs=-+
  Switch1 : Switch  Criteria=u2 > Threshold  Threshold=0.3  ZeroCross=off
  "d " : InportShadow  Port=3
  dsPIC_ABS : SLUGS_Library/dsPIC_ABS
  dsPIC_ABS1 : SLUGS_Library/dsPIC_ABS
  dsPIC_SQRT : SLUGS_Library/dsPIC_SQRT
  negprotect1 : MATLAB Function  TreatAsAtomicUnit=on
  negprotect2 : MATLAB Function  TreatAsAtomicUnit=on
  L2 Vec : Outport
  Mode : Outport  Port=2
  wires:
  R/1 -> Product/1, Product/2
  L2/1 -> Product1/1, Product1/2
  d/1 -> Product2/1, Product2/2, Subtract1/1, Subtract1/2
  Product/1 -> Subtract/1, Subtract2/1  "r^2"
  Product1/1 -> Subtract/2
  Product2/1 -> Subtract/3
  Subtract/1 -> Product3/1  "r^2 - L2^2 + d^2"
  negprotect2/1(zpVal) -> Product3/2  "2d"
  Subtract1/1 -> negprotect2/1(val)
  Product3/1 -> Product4/2, Product4/1, [a]  "a"
  Product4/1 -> Subtract2/2  "a^2"
  Subtract2/1 -> dsPIC_SQRT/1  "h"
  negprotect1/1(zpVal) -> Product6/2  "d"
  "d "/1 -> negprotect1/1(val)
  ISR Loc/1 -> Subtract3/1
  Subtract3/1 -> Embedded MATLAB Function/2(P2)  "P2"
  UAV m ISR/1 -> Product6/1
  Product7/1 -> Subtract3/2
  Product6/1 -> Product7/1, [UavMIsDbd]
  [a] -> Product7/2
  [UavMIsDbd] -> Product5/2
  Vxyz/1 -> Compute Angle Between Vectors1/1, Compute Angle Between Vectors2/1
  |Vg|/1 -> Compute Angle Between Vectors1/2, Compute Angle Between Vectors2/2
  Compute Angle Between Vectors2/1 -> dsPIC_ABS1/1
  dsPIC_ABS1/1 -> Relational Operator/1
  Compute Angle Between Vectors1/1 -> dsPIC_ABS/1
  dsPIC_ABS/1 -> Relational Operator/2
  Relational Operator/1 -> Switch1/2
  RTB1/1 -> Mode/1
  dsPIC_SQRT/1 -> Product5/1  "h"
  Product5/1 -> Embedded MATLAB Function/1(hFact)
  Subtract5/1 -> Compute Angle Between Vectors2/3, Switch1/1
  Embedded MATLAB Function/1(P31) -> Subtract5/1
  Subtract6/1 -> Compute Angle Between Vectors1/3, Switch1/3
  Embedded MATLAB Function/2(P32) -> Subtract6/2
  Puav/1 -> Subtract5/2, Subtract6/1
  Switch1/1 -> L2 Vec/1

== system InnerOuter_Sim_newNav_flightgear_L2/Navigation/Circle Navigation/No intersection,  Navigate to ISR ==
  Puav : Inport
  ISR Loc : Inport  Port=2
  Action Port : ActionPort  ActionType=then
  RTB1 : Constant  Value=0  OutDataTypeStr=uint8
  Subtract : Sum  Inputs=+-
  L2 Vec : Outport
  Mode : Outport  Port=2
  wires:
  ISR Loc/1 -> Subtract/1
  Puav/1 -> Subtract/2
  Subtract/1 -> L2 Vec/1
  RTB1/1 -> Mode/1

== system InnerOuter_Sim_newNav_flightgear_L2/Navigation/L2+/Get Sin, Cos eta ==
  |V_g| : Inport
  L2_vec : Inport  Port=2
  Vxyz : Inport  Port=3
  "2D Dot Product " : Subsystem
  Compare To Zero : simulink/Logic and Bit Operations/Compare To Zero  relop===  OutDataTypeStr=uint8  ZeroCross=off
  Dead Zone : DeadZone  LowerValue=-0.1  UpperValue=0.1  SaturateOnIntegerOverflow=on
  Display : Display
  Display1 : Display
  Divide1 : Product  Inputs=/*
  Divide2 : Product  Inputs=*/
  Get  Groundspeed : Subsystem
  Get ZProd : Subsystem
  Product1 : Product  RndMeth=Zero
  Switch : Switch  Criteria=u2 > Threshold  Threshold=0.3  ZeroCross=off
  Switch2 : Switch  Criteria=u2 > Threshold  Threshold=0.3  ZeroCross=off
  cos(pi/2) : Constant  Value=0  OutDataTypeStr=single
  negprotect : MATLAB Function  TreatAsAtomicUnit=on
  sin(pi/2) : Constant  OutDataTypeStr=single
  sin(eta) : Outport
  cos(eta) : Outport  Port=2
  wires:
  negprotect/1(zpVal) -> Divide2/2, Divide1/1, Dead Zone/1
  Switch/1 -> Display/1, sin(eta)/1
  Divide2/1 -> Switch/3
  Get ZProd/1(Z_prod) -> Divide2/1
  Divide1/1 -> Switch2/3
  cos(pi/2)/1 -> Switch2/1
  Switch2/1 -> Display1/1, cos(eta)/1
  sin(pi/2)/1 -> Switch/1
  "2D Dot Product "/1(2D _dot) -> Divide1/2
  Product1/1 -> negprotect/1(val)
  |V_g|/1 -> Product1/2
  Get  Groundspeed/1(|L2|) -> Product1/1
  Vxyz/1 -> "2D Dot Product "/1(Vxyz), Get ZProd/2(Vxyz)
  L2_vec/1 -> Get  Groundspeed/1(L2_vec), "2D Dot Product "/2(L2_vec), Get ZProd/1(L2_vec)
  Dead Zone/1 -> Compare To Zero/1
  Compare To Zero/1 -> Switch2/2, Switch/2

== system InnerOuter_Sim_newNav_flightgear_L2/Navigation/L2+/L2+ ==
  sin(eta) : Inport
  |V_g| : Inport  Port=2
  T* : Inport  Port=3
  Display3 : Display
  Divide : Product  Inputs=**/
  Gain : Gain  Gain=2  SampleTime=0.01
  negprotect : MATLAB Function  TreatAsAtomicUnit=on
  a_c : Outport
  wires:
  T*/1 -> negprotect/1(val)
  Gain/1 -> Display3/1, a_c/1
  |V_g|/1 -> Divide/2
  Divide/1 -> Gain/1
  sin(eta)/1 -> Divide/1
  negprotect/1(zpVal) -> Divide/3

== system InnerOuter_Sim_newNav_flightgear_L2/Navigation/L2+/Subsystem ==
  a_c : Inport
  Bank  Limit Command : Saturate  UpperLimit=bankCommandLimit  LowerLimit=-bankCommandLimit  SampleTime=apSampleTime
  Constant : Constant  Value=ISA_g  OutDataTypeStr=single
  Product : Product  Inputs=*/  RndMeth=Zero
  To Workspace3 : ToWorkspace  VariableName=Phic  SampleTime=-1  SaveFormat=Array
  dsPIC_atan : SLUGS_Library/dsPIC_atan
  phi_c : Outport
  wires:
  Bank  Limit Command/1 -> To Workspace3/1, phi_c/1
  dsPIC_atan/1 -> Bank  Limit Command/1
  Product/1 -> dsPIC_atan/1
  Constant/1 -> Product/2
  a_c/1 -> Product/1

== system InnerOuter_Sim_newNav_flightgear_L2/Navigation/L2+/if sin(eta) < 0 - maxAcc else                 maxAcc  ==
  sin(eta) : Inport
  Compare To Zero : simulink/Logic and Bit Operations/Compare To Zero  relop=<  OutDataTypeStr=uint8  ZeroCross=off
  Constant1 : Constant  Value=maxAcc  OutDataTypeStr=single
  Constant9 : Constant  Value=-maxAcc  OutDataTypeStr=single
  Switch1 : Switch  Criteria=u2 > Threshold  Threshold=0.3
  + - maxAcc : Outport
  wires:
  Switch1/1 -> + - maxAcc/1
  sin(eta)/1 -> Compare To Zero/1
  Constant1/1 -> Switch1/3
  Constant9/1 -> Switch1/1
  Compare To Zero/1 -> Switch1/2

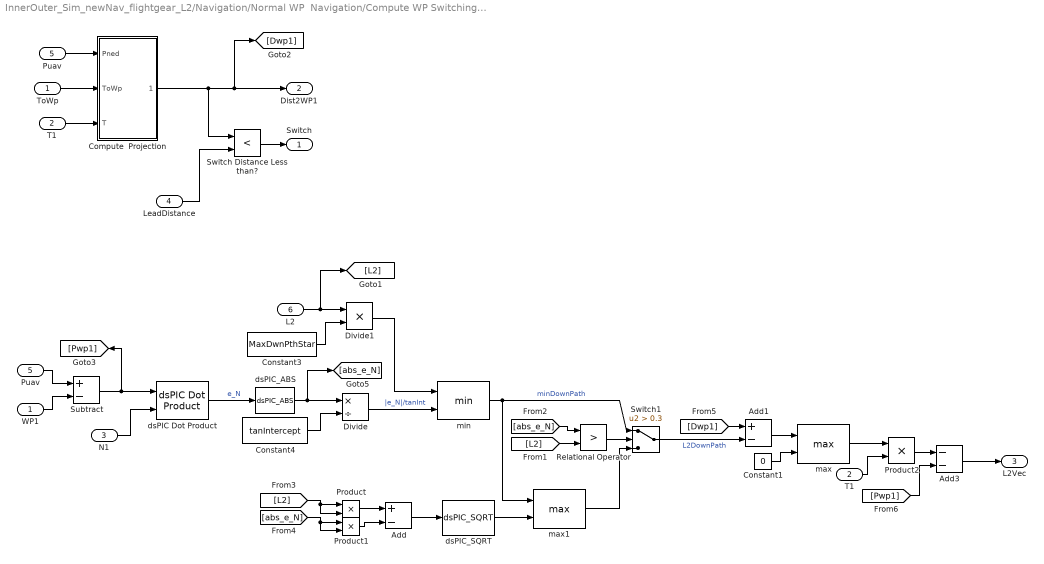
== system InnerOuter_Sim_newNav_flightgear_L2/Navigation/Normal WP  Navigation/Compute WP Switching Trigger ==
  ToWp : Inport
  T1 : Inport  Port=2
  N1 : Inport  Port=3
  LeadDistance : Inport  Port=4
  Puav : Inport  Port=5
  L2 : Inport  Port=6
  Add : Sum  Inputs=+-
  Add1 : Sum  Inputs=+-
  Add3 : Sum  Inputs=--
  Compute  Projection : Subsystem
  Constant1 : Constant  Value=0  OutDataTypeStr=single
  Constant3 : Constant  Value=MaxDwnPthStar  OutDataTypeStr=single
  Constant4 : Constant  Value=tanIntercept  OutDataTypeStr=single
  Divide : Product  Inputs=*/
  Divide1 : Product
  Product : Product  RndMeth=Zero
  Product1 : Product  RndMeth=Zero
  Product2 : Product  RndMeth=Zero
  "Puav " : InportShadow  Port=5
  Relational Operator : RelationalOperator  Operator=>  OutDataTypeStr=boolean
  Subtract : Sum  Inputs=+-  OutDataTypeStr=single
  Switch Distance Less than? : RelationalOperator  Operator=<  OutDataTypeStr=uint(8)  SampleTime=apSampleTime
  Switch1 : Switch  Criteria=u2 > Threshold  Threshold=0.3
  "T1 " : InportShadow  Port=2
  "WP1 " : InportShadow  Port=1
  dsPIC Dot Product : SLUGS_Library/dsPIC Dot Product
  dsPIC_ABS : SLUGS_Library/dsPIC_ABS
  dsPIC_SQRT : SLUGS_Library/dsPIC_SQRT
  max : SLUGS_Library/max
  max1 : SLUGS_Library/max
  min : SLUGS_Library/min
  Switch : Outport
  Dist2WP1 : Outport  Port=2
  L2Vec : Outport  Port=3
  wires:
  Puav/1 -> Compute  Projection/1(Pned)
  Compute  Projection/1(D2wp1) -> Switch Distance Less than?/1, Dist2WP1/1, [Dwp1]
  LeadDistance/1 -> Switch Distance Less than?/2
  ToWp/1 -> Compute  Projection/2(ToWp)
  T1/1 -> Compute  Projection/3(T)
  Switch Distance Less than?/1 -> Switch/1
  "Puav "/1 -> Subtract/1
  "WP1 "/1 -> Subtract/2
  Subtract/1 -> dsPIC Dot Product/1, [Pwp1]
  dsPIC Dot Product/1 -> dsPIC_ABS/1  "e_N"
  dsPIC_ABS/1 -> Divide/1, [abs_e_N]
  Constant4/1 -> Divide/2
  Divide/1 -> min/2  "|e_N|/tanInt"
  L2/1 -> Divide1/1, [L2]
  Constant3/1 -> Divide1/2
  Divide1/1 -> min/1
  min/1 -> max1/1, Switch1/1  "minDownPath"
  Relational Operator/1 -> Switch1/2
  [L2] -> Relational Operator/2
  [abs_e_N] -> Relational Operator/1
  Switch1/1 -> Add1/2  "L2DownPath"
  Add/1 -> dsPIC_SQRT/1
  dsPIC_SQRT/1 -> max1/2
  [L2] -> Product/1, Product/2
  Product/1 -> Add/1
  [abs_e_N] -> Product1/2, Product1/1
  Product1/1 -> Add/2
  max1/1 -> Switch1/3
  [Dwp1] -> Add1/1
  Add1/1 -> max/1
  Constant1/1 -> max/2
  max/1 -> Product2/1
  "T1 "/1 -> Product2/2
  Product2/1 -> Add3/1
  [Pwp1] -> Add3/2
  Add3/1 -> L2Vec/1
  N1/1 -> dsPIC Dot Product/2

== system InnerOuter_Sim_newNav_flightgear_L2/Navigation/Normal WP  Navigation/Get Frenet ==
  GS LLA : Inport
  GS R_in : Inport  Port=2
  From WP : Inport  Port=3
  To WP : Inport  Port=4
  TurnLeadTime : Inport  Port=5
  |V_g| : Inport  Port=6
  Enable : EnablePort
  Compute Frenet : SLUGS_Library/Navigation/Compute Frenet
  Demux1 : Demux  Outputs=3
  Display : Display
  GS LLA_1 : InportShadow  Port=1
  GS R_in_1 : InportShadow  Port=2
  Integer Delay1 : Delay  DelayLength=1  InitialCondition=1  InputProcessing=Inherited
  Log 2 [navSupport.c] : dsPICdrivers/OTHERS/C Function Call  Tag=dsPIC_dsPIC_CFunctionCall  FctUpdate=Output Function  fctName='setLogFloat2'  INPUT_SIZE=3  INPUT1=real32  INPUT2=--  INPUT3=--  OUTPUT_SIZE=1  OUTPUT1=--  SampleTime=.01  InputType=[ 7 ]  OutputType=[ ]  FctDeclaration=extern void setLogFloat2(real32_T* u1);  FctCall=setLogFloat2(*%u1);  OrderingInOutPopup=None  FctStart=None  FctStart_Name=Init_onlyOnce  FctStart_Declaration=inline extern void Init_onlyOnce();  FctStart_Call=Init_onlyOnce();  FctInit=None  FctInit_Name=Init_Reset  FctInit_Declaration=inline extern void Init_Reset();  FctInit_Call=Init_Reset();  PinDigitalInput=[]  PinDigitalOutput=[]  AnalogueInput=[]
  Product1 : Product  OutDataTypeStr=single  RndMeth=Zero
  To Workspace2 : ToWorkspace  VariableName=fromWP  SampleTime=-1  SaveFormat=Array
  To Workspace3 : ToWorkspace  VariableName=toWP  SampleTime=-1  SaveFormat=Array
  Zero out Z1 : MATLAB Function  TreatAsAtomicUnit=on
  Zero out Z2 : MATLAB Function  TreatAsAtomicUnit=on
  Zero out Z3 : MATLAB Function  TreatAsAtomicUnit=on
  get WP Coord from Index1 : SLUGS_Library/Navigation/get WP Coord from Index
  get WP Coord from Index2 : Subsystem  AncestorBlock=SLUGS_Library/Navigation/get WP Coord from Index
  H_c : Outport
  ToWp : Outport  Port=2
  T1 : Outport  Port=3
  N1 : Outport  Port=4
  TurnLeadDistance : Outport  Port=5
  wires:
  Zero out Z3/1(P) -> ToWp/1
  Integer Delay1/1 -> H_c/1
  Compute Frenet/2 -> Zero out Z1/1(Pin)
  Demux1/3 -> Integer Delay1/1, Display/1
  Compute Frenet/1 -> Zero out Z2/1(Pin)
  |V_g|/1 -> Product1/2
  TurnLeadTime/1 -> Product1/1
  Product1/1 -> TurnLeadDistance/1
  Zero out Z2/1(P) -> T1/1
  Zero out Z1/1(P) -> N1/1
  get WP Coord from Index1/1 -> Log 2 [navSupport.c]/1, Compute Frenet/1, To Workspace2/1
  get WP Coord from Index2/1(WP Coord) -> Compute Frenet/2, To Workspace3/1, Zero out Z3/1(Pin), Demux1/1
  From WP/1 -> get WP Coord from Index1/1
  GS LLA/1 -> get WP Coord from Index1/2
  GS R_in/1 -> get WP Coord from Index1/3
  To WP/1 -> get WP Coord from Index2/1(WP Idx)
  GS LLA_1/1 -> get WP Coord from Index2/2(GS LLA)
  GS R_in_1/1 -> get WP Coord from Index2/3(GS R_in)

== system InnerOuter_Sim_newNav_flightgear_L2/Navigation/Normal WP  Navigation/On WP Enable ==
  L2 : Inport
  GS LLA : Inport  Port=2
  GS R_in : Inport  Port=3
  Enable : EnablePort
  Constant5 : Constant  Value=IPStar  OutDataTypeStr=single
  Product : Product  Inputs=3  RndMeth=Zero
  Subsystem : Subsystem
  Subtract : Sum  Inputs=+-
  P_i : Outport
  wires:
  Constant5/1 -> Product/3
  L2/1 -> Product/1
  Product/1 -> Subtract/2
  Subtract/1 -> P_i/1  "WP0 - L2*IP*T1"
  GS LLA/1 -> Subsystem/1(GS LLA)
  GS R_in/1 -> Subsystem/2(GS R_in)
  Subsystem/2(T1) -> Product/2
  Subsystem/1(WP0) -> Subtract/1

== system InnerOuter_Sim_newNav_flightgear_L2/Navigation/Normal WP  Navigation/Subsystem ==
  DidReachIP : Inport
  Data Type Conversion3 : DataTypeConversion  OutDataTypeStr=uint8  SampleTime=apSampleTime
  Detect Rising Transition [navSupport.c] : dsPICdrivers/OTHERS/C Function Call  Tag=dsPIC_dsPIC_CFunctionCall  FctUpdate=Output Function  fctName='justEnabled'  INPUT_SIZE=1  INPUT1=uint8  INPUT2=uint8  INPUT3=--  OUTPUT_SIZE=1  OUTPUT1=uint8  SampleTime=0.01  InputType=[ 2 2 ]  OutputType=[ 2 ]  FctDeclaration=extern uint8_T justEnabled(uint8_T u1, uint8_T u2);  FctCall=%y1 = justEnabled(%u1, %u2);  OrderingInOutPopup=None  FctStart=None  FctStart_Name=Init_onlyOnce  FctStart_Declaration=inline extern void Init_onlyOnce();  FctStart_Call=Init_onlyOnce();  FctInit=None  FctInit_Name=Init_Reset  FctInit_Declaration=inline extern void Init_Reset();  FctInit_Call=Init_Reset();  PinDigitalInput=[]  PinDigitalOutput=[]  AnalogueInput=[]
  Index : Constant  OutDataTypeStr=uint8
  Just Enab : Outport
  wires:
  Index/1 -> Detect Rising Transition [navSupport.c]/2
  DidReachIP/1 -> Data Type Conversion3/1
  Detect Rising Transition [navSupport.c]/1 -> Just Enab/1
  Data Type Conversion3/1 -> Detect Rising Transition [navSupport.c]/1

== system InnerOuter_Sim_newNav_flightgear_L2/Navigation/RTB/Follow Mobile Navigation/Compute Mobile Location ==
  "Lat, Lon" : Inport
  GS LLA : Inport  Port=2
  GS R : Inport  Port=3
  Enable : EnablePort  StatesWhenEnabling=reset
  Demux4 : Demux  Outputs=2
  Geod2LTP : SLUGS_Library/Navigation/Geod2LTP
  No Height All in 2D : Constant  Value=0  OutDataTypeStr=single
  XYZ : Outport
  wires:
  Geod2LTP/1 -> XYZ/1
  "Lat, Lon"/1 -> Demux4/1
  Demux4/2 -> Geod2LTP/4
  Demux4/1 -> Geod2LTP/3
  No Height All in 2D/1 -> Geod2LTP/5
  GS R/1 -> Geod2LTP/2
  GS LLA/1 -> Geod2LTP/1

== system InnerOuter_Sim_newNav_flightgear_L2/Navigation/RTB/Follow Mobile Navigation/Simple Predictor ==
  Base Point : Inport
  Discrete-Time Integrator : DiscreteIntegrator  InitialConditionSource=external  SampleTime=-1  ICPrevOutput=DiscIntNeverNeededParam  ICPrevScaledInput=DiscIntNeverNeededParam
  Gain : Gain
  Gain1 : Gain  Gain=3
  Sum : Sum  Inputs=|+-
  Sum1 : Sum  Inputs=++|
  Predicted Bp : Outport
  wires:
  Discrete-Time Integrator/1 -> Gain/1
  Sum/1 -> Gain1/1, Discrete-Time Integrator/1
  Gain/1 -> Sum/2, Sum1/2
  Gain1/1 -> Sum1/1
  Base Point/1 -> Sum/1, Discrete-Time Integrator/2
  Sum1/1 -> Predicted Bp/1

== system InnerOuter_Sim_newNav_flightgear_L2/Navigation/Recent Enable/Grab Upon Enable ==
  Enable : EnablePort
  Compute GS Location : Subsystem
  Constant : Constant  Value=GS_location  OutDataTypeStr=single
  Data Type Conversion : DataTypeConversion  OutDataTypeStr=single
  Data Type Conversion1 : DataTypeConversion  OutDataTypeStr=single
  Demux : Demux  Outputs=[1 2]
  Demux1 : Demux  Outputs=3
  Display6 : Display
  Display7 : Display
  Display8 : Display
  Environment Controller : simulink/Signal Routing/Environment Controller
  Get the GS Location [updateControlMCUState.c] : dsPICdrivers/OTHERS/C Function Call  Tag=dsPIC_dsPIC_CFunctionCall  FctUpdate=Output Function  fctName='getGSLocation'  INPUT_SIZE=1  INPUT1=--  INPUT2=--  INPUT3=--  OUTPUT_SIZE=3  OUTPUT1=real32  SampleTime=0.01  InputType=[ ]  OutputType=[ 7 ]  FctDeclaration=extern void getGSLocation(real32_T* y1);  FctCall=getGSLocation(*%y1);  OrderingInOutPopup=None  FctStart=None  FctStart_Name=Init_onlyOnce  FctStart_Declaration=inline extern void Init_onlyOnce();  FctStart_Call=Init_onlyOnce();  FctInit=None  FctInit_Name=Init_Reset  FctInit_Declaration=inline extern void Init_Reset();  FctInit_Call=Init_Reset();  PinDigitalInput=[]  PinDigitalOutput=[]  AnalogueInput=[]
  Terminator : Terminator
  "GS, Lon, Lat" : Outport
  GS R_in : Outport  Port=2
  GS Altitude (m) : Outport  Port=3
  wires:
  Demux/2 -> Terminator/1
  Demux/1 -> GS Altitude (m)/1
  Compute GS Location/2(R_in) -> Data Type Conversion1/1, Demux1/1
  Compute GS Location/1("Lon, Lat") -> Data Type Conversion/1
  Data Type Conversion/1 -> "GS, Lon, Lat"/1
  Data Type Conversion1/1 -> GS R_in/1
  Constant/1 -> Environment Controller/1
  Get the GS Location [updateControlMCUState.c]/1 -> Environment Controller/2
  Environment Controller/1 -> Compute GS Location/1(GS Location), Demux/1
  Demux1/1 -> Display6/1
  Demux1/2 -> Display7/1
  Demux1/3 -> Display8/1
